simulink model "speed_estimator_pll_model"  (R2023b)
settings: Solver=FixedStepDiscrete  StartTime=0.0  StopTime=0.010  FixedStep=5e-05  RelTol=1e-3
values from neighbouring files (symbols this model uses):
  EncoderOffsetRad = 0.0    [speed_estimator_pll_interface.sldd]
  InvGearRatio = 0.0054540494456887245    [speed_estimator_pll_interface.sldd]
  PllKi = 5116403.0    [speed_estimator_pll_interface.sldd]
  PllKp = 4523.8935546875    [speed_estimator_pll_interface.sldd]
  PolePairs = 2.0    [speed_estimator_pll_interface.sldd]
  SpeedEstimatorSampleTime = 4.9999998736893758E-5    [speed_estimator_pll_interface.sldd]
  ZeroSpeedThresholdRadS = 0.012263224460184574    [speed_estimator_pll_interface.sldd]
settings Model: DataDictionary=speed_estimator_pll_interface.sldd  Creator=user  LastModifiedBy=user
settings OptimizationCC: EnhancedBackFolding=on  PassReuseOutputArgsAs=Individual arguments  OptimizeBlockOrder=speed  DifferentSizesBufferReuse=on  OptimizationCustomize=off  EfficientTunableParamExpr=on
settings DebuggingCC: ParameterPrecisionLossMsg=none  ParameterTunabilityLossMsg=error
settings HardwareCC: ProdBitPerPointer=32  ProdBitPerSizeT=32  ProdBitPerPtrDiffT=32  ProdLargestAtomicInteger=Long  ProdLargestAtomicFloat=Double  ProdWordSize=32  ProdHWDeviceType=ARM Compatible->ARM Cortex  TargetLargestAtomicInteger=Long  TargetLargestAtomicFloat=Double  TargetIntDivRoundTo=Zero  TargetEndianess=LittleEndian  TargetHWDeviceType=ARM Compatible->ARM Cortex  ProdEqTarget=off
settings SFSimCC: MATLABDynamicMemAlloc=off
settings RTWCC: Description=Embedded Coder  SystemTargetFile=ert.tlc  GenCodeOnly=on  TemplateMakefile=ert_default_tmf  GenerateReport=on
settings CodeAppCC: ForceParamTrailComments=on  IgnoreCustomStorageClasses=off  OperatorAnnotations=on  SimulinkDataObjDesc=on  SFDataObjDesc=on  InsertBlockDesc=on
settings ERTTargetCC: TargetLangStandard=C99 (ISO)  CodeInterfacePackaging=Reusable function  ERTCustomFileTemplate=example_file_process.tlc

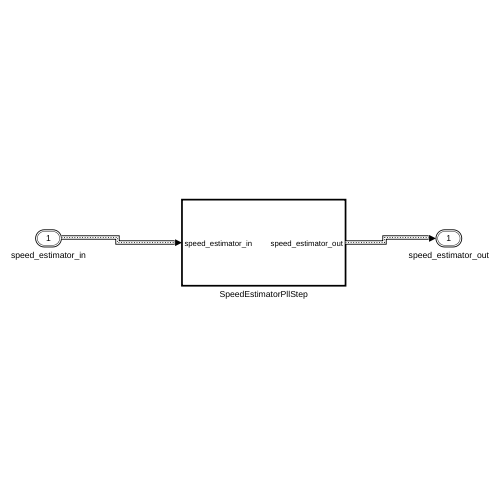
[thumbnail: Simulink's stored preview of the top-level diagram]
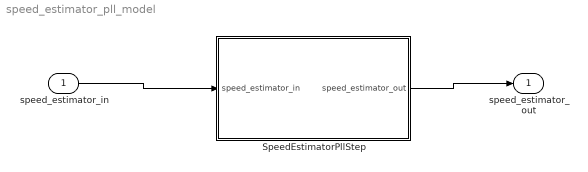
== system speed_estimator_pll_model ==
  speed_estimator_in : Inport  OutDataTypeStr=Bus: speed_estimator_input_t  SampleTime=50e-6  BusOutputAsStruct=on
  SpeedEstimatorPllStep : Subsystem  TreatAsAtomicUnit=on  RTWFcnName=SpeedEstimatorPllStep  RTWFileName=SpeedEstimatorPllStep
      settings: RTWFcnNameOpts=User specified  RTWFileNameOpts=User specified
  speed_estimator_out : Outport  OutDataTypeStr=Bus: speed_estimator_output_t
  wires:
  speed_estimator_in/1 -> SpeedEstimatorPllStep/1(speed_estimator_in)
  SpeedEstimatorPllStep/1(speed_estimator_out) -> speed_estimator_out/1

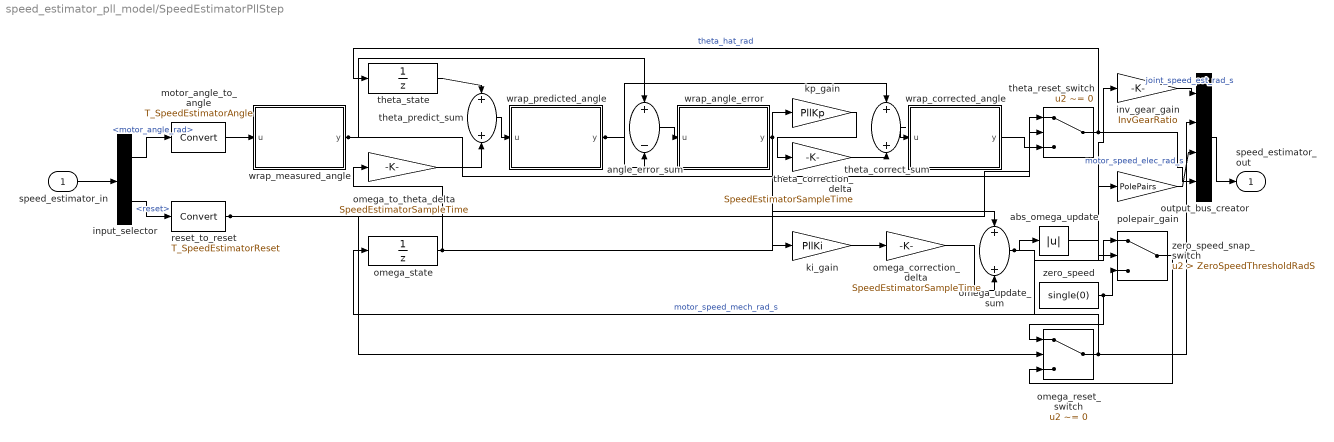
== system speed_estimator_pll_model/SpeedEstimatorPllStep ==
  speed_estimator_in : Inport  OutDataTypeStr=Bus: speed_estimator_input_t  BusOutputAsStruct=on
  abs_omega_update : Abs  SaturateOnIntegerOverflow=off
  angle_error_sum : Sum  Inputs=+-  OutDataTypeStr=T_SpeedEstimatorAngle  AccumDataTypeStr=T_SpeedEstimatorAngle
  input_selector : BusSelector  OutputSignals=motor_angle_rad,reset
  inv_gear_gain : Gain  Gain=InvGearRatio  ParamDataTypeStr=T_SpeedEstimatorGain  OutDataTypeStr=T_SpeedEstimatorSpeed
  ki_gain : Gain  Gain=PllKi  ParamDataTypeStr=T_SpeedEstimatorGain  OutDataTypeStr=T_SpeedEstimatorSpeed
  kp_gain : Gain  Gain=PllKp  ParamDataTypeStr=T_SpeedEstimatorGain  OutDataTypeStr=T_SpeedEstimatorAngle
  motor_angle_to_angle : DataTypeConversion  OutDataTypeStr=T_SpeedEstimatorAngle  SaturateOnIntegerOverflow=off  RndMeth=Floor
  omega_correction_delta : Gain  Gain=SpeedEstimatorSampleTime  ParamDataTypeStr=T_SpeedEstimatorFloat  OutDataTypeStr=T_SpeedEstimatorSpeed
  omega_reset_switch : Switch  Criteria=u2 ~= 0  SaturateOnIntegerOverflow=off  InputSameDT=off
  omega_state : UnitDelay  SampleTime=50e-6  HasFrameUpgradeWarning=on
  omega_to_theta_delta : Gain  Gain=SpeedEstimatorSampleTime  ParamDataTypeStr=T_SpeedEstimatorFloat  OutDataTypeStr=T_SpeedEstimatorAngle
  omega_update_sum : Sum  OutDataTypeStr=T_SpeedEstimatorSpeed  AccumDataTypeStr=T_SpeedEstimatorSpeed
  output_bus_creator : BusCreator  Inputs=4  OutDataTypeStr=Bus: speed_estimator_output_t  NonVirtualBus=on
  polepair_gain : Gain  Gain=PolePairs  ParamDataTypeStr=T_SpeedEstimatorGain  OutDataTypeStr=T_SpeedEstimatorSpeed
  reset_to_reset : DataTypeConversion  OutDataTypeStr=T_SpeedEstimatorReset  SaturateOnIntegerOverflow=off  RndMeth=Floor
  theta_correct_sum : Sum  OutDataTypeStr=T_SpeedEstimatorAngle  AccumDataTypeStr=T_SpeedEstimatorAngle
  theta_correction_delta : Gain  Gain=SpeedEstimatorSampleTime  ParamDataTypeStr=T_SpeedEstimatorFloat  OutDataTypeStr=T_SpeedEstimatorAngle
  theta_predict_sum : Sum  OutDataTypeStr=T_SpeedEstimatorAngle  AccumDataTypeStr=T_SpeedEstimatorAngle
  theta_reset_switch : Switch  Criteria=u2 ~= 0  SaturateOnIntegerOverflow=off  InputSameDT=off
  theta_state : UnitDelay  InitialCondition=EncoderOffsetRad  SampleTime=50e-6  HasFrameUpgradeWarning=on
  wrap_angle_error : Subsystem
  wrap_corrected_angle : Subsystem
  wrap_measured_angle : Subsystem
  wrap_predicted_angle : Subsystem
  zero_speed : Constant  Value=single(0)  OutDataTypeStr=T_SpeedEstimatorSpeed  SampleTime=50e-6
  zero_speed_snap_switch : Switch  Criteria=u2 > Threshold  Threshold=ZeroSpeedThresholdRadS  SaturateOnIntegerOverflow=off  InputSameDT=off
  speed_estimator_out : Outport  OutDataTypeStr=Bus: speed_estimator_output_t
  wires:
  speed_estimator_in/1 -> input_selector/1
  input_selector/1 -> motor_angle_to_angle/1  "<motor_angle_rad>"
  input_selector/2 -> reset_to_reset/1  "<reset>"
  motor_angle_to_angle/1 -> wrap_measured_angle/1(u)
  theta_state/1 -> theta_predict_sum/1
  omega_state/1 -> omega_to_theta_delta/1, omega_update_sum/1
  omega_to_theta_delta/1 -> theta_predict_sum/2
  theta_predict_sum/1 -> wrap_predicted_angle/1(u)
  wrap_measured_angle/1(y) -> angle_error_sum/1, theta_reset_switch/1
  wrap_predicted_angle/1(y) -> angle_error_sum/2, theta_correct_sum/1
  angle_error_sum/1 -> wrap_angle_error/1(u)
  wrap_angle_error/1(y) -> kp_gain/1, ki_gain/1
  kp_gain/1 -> theta_correction_delta/1
  theta_correction_delta/1 -> theta_correct_sum/2
  theta_correct_sum/1 -> wrap_corrected_angle/1(u)
  ki_gain/1 -> omega_correction_delta/1
  omega_correction_delta/1 -> omega_update_sum/2
  omega_update_sum/1 -> abs_omega_update/1, zero_speed_snap_switch/1
  abs_omega_update/1 -> zero_speed_snap_switch/2
  zero_speed/1 -> zero_speed_snap_switch/3, omega_reset_switch/1
  reset_to_reset/1 -> omega_reset_switch/2, theta_reset_switch/2
  zero_speed_snap_switch/1 -> omega_reset_switch/3
  wrap_corrected_angle/1(y) -> theta_reset_switch/3
  omega_reset_switch/1 -> omega_state/1, inv_gear_gain/1, polepair_gain/1, output_bus_creator/2  "motor_speed_mech_rad_s"
  theta_reset_switch/1 -> theta_state/1, output_bus_creator/4  "theta_hat_rad"
  inv_gear_gain/1 -> output_bus_creator/1  "joint_speed_est_rad_s"
  polepair_gain/1 -> output_bus_creator/3  "motor_speed_elec_rad_s"
  output_bus_creator/1 -> speed_estimator_out/1

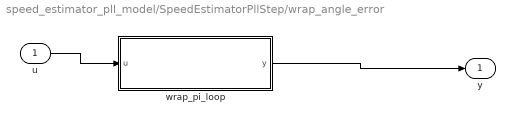
== system speed_estimator_pll_model/SpeedEstimatorPllStep/wrap_angle_error ==
  u : Inport  OutDataTypeStr=T_SpeedEstimatorAngle
  wrap_pi_loop : MATLAB Function  TreatAsAtomicUnit=on
  y : Outport  OutDataTypeStr=T_SpeedEstimatorAngle
  wires:
  u/1 -> wrap_pi_loop/1(u)
  wrap_pi_loop/1(y) -> y/1

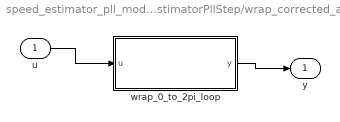
== system speed_estimator_pll_model/SpeedEstimatorPllStep/wrap_corrected_angle ==
  u : Inport  OutDataTypeStr=T_SpeedEstimatorAngle
  wrap_0_to_2pi_loop : MATLAB Function  TreatAsAtomicUnit=on
  y : Outport  OutDataTypeStr=T_SpeedEstimatorAngle
  wires:
  u/1 -> wrap_0_to_2pi_loop/1(u)
  wrap_0_to_2pi_loop/1(y) -> y/1

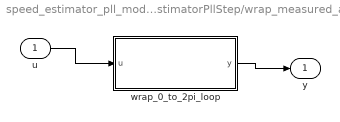
== system speed_estimator_pll_model/SpeedEstimatorPllStep/wrap_measured_angle ==
  u : Inport  OutDataTypeStr=T_SpeedEstimatorAngle
  wrap_0_to_2pi_loop : MATLAB Function  TreatAsAtomicUnit=on
  y : Outport  OutDataTypeStr=T_SpeedEstimatorAngle
  wires:
  u/1 -> wrap_0_to_2pi_loop/1(u)
  wrap_0_to_2pi_loop/1(y) -> y/1

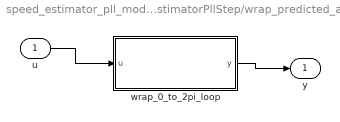
== system speed_estimator_pll_model/SpeedEstimatorPllStep/wrap_predicted_angle ==
  u : Inport  OutDataTypeStr=T_SpeedEstimatorAngle
  wrap_0_to_2pi_loop : MATLAB Function  TreatAsAtomicUnit=on
  y : Outport  OutDataTypeStr=T_SpeedEstimatorAngle
  wires:
  u/1 -> wrap_0_to_2pi_loop/1(u)
  wrap_0_to_2pi_loop/1(y) -> y/1

== matlab function speed_estimator_pll_model/SpeedEstimatorPllStep/wrap_measured_angle/wrap_0_to_2pi_loop ==
  data: u input; y output
function y = wrap_0_to_2pi_loop(u)
%#codegen
two_pi = single(6.2831853071795864769);
y = single(u);
while y >= two_pi
    y = y - two_pi;
end
while y < single(0.0)
    y = y + two_pi;
end
end

== matlab function speed_estimator_pll_model/SpeedEstimatorPllStep/wrap_angle_error/wrap_pi_loop ==
  data: u input; y output
function y = wrap_pi_loop(u)
%#codegen
pi_v = single(3.1415926535897932385);
y = wrap_0_to_2pi_loop(single(u) + pi_v) - pi_v;
end

function y = wrap_0_to_2pi_loop(u)
%#codegen
two_pi = single(6.2831853071795864769);
y = single(u);
while y >= two_pi
    y = y - two_pi;
end
while y < single(0.0)
    y = y + two_pi;
end
end

== matlab function speed_estimator_pll_model/SpeedEstimatorPllStep/wrap_corrected_angle/wrap_0_to_2pi_loop ==
  data: u input; y output
function y = wrap_0_to_2pi_loop(u)
%#codegen
two_pi = single(6.2831853071795864769);
y = single(u);
while y >= two_pi
    y = y - two_pi;
end
while y < single(0.0)
    y = y + two_pi;
end
end

== matlab function speed_estimator_pll_model/SpeedEstimatorPllStep/wrap_predicted_angle/wrap_0_to_2pi_loop ==
  data: u input; y output
function y = wrap_0_to_2pi_loop(u)
%#codegen
two_pi = single(6.2831853071795864769);
y = single(u);
while y >= two_pi
    y = y - two_pi;
end
while y < single(0.0)
    y = y + two_pi;
end
end
